simulink model "scalar_processor"  (Simulink 7.4)
settings: Solver=ode45  StartTime=0.0  StopTime=10.0  RelTol=1e-3
undefined symbols (not defined in the file): AS_ABS, CT_NONE, CT_S32, CT_U32
libraries: xbsIndex_r4 x517
(part 1 of 3)
settings Model: Creator=andryc  LastModifiedBy=andryc

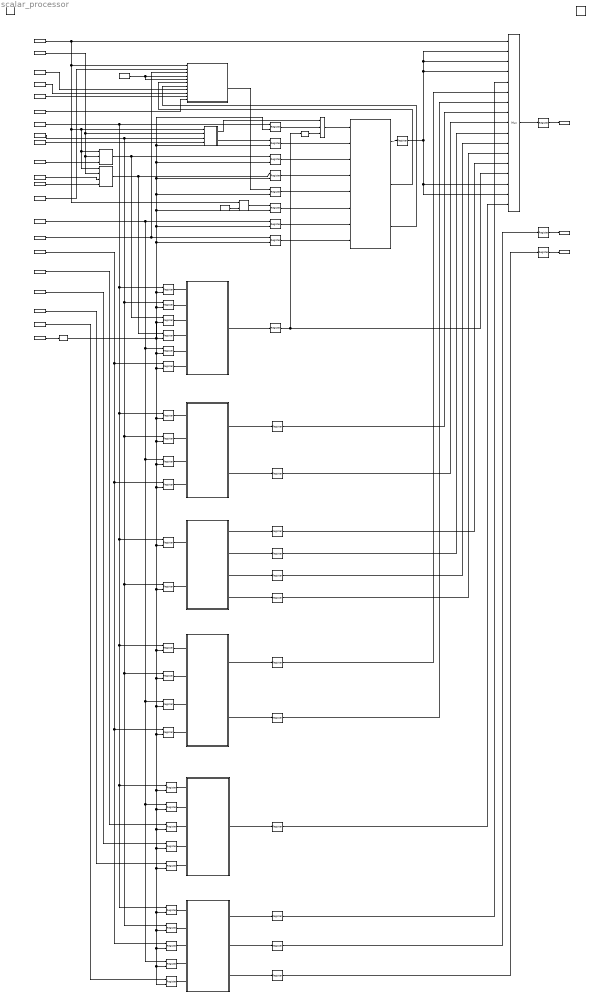
== system scalar_processor ==
  " System Generator" : xbsIndex_r4/ System Generator  Tag=genX  SystemSampleTime=-1  xilinxfamily=virtex5  part=xc5vlx50t  speed=-1  package=ff1136  synthesis_tool=XST  clock_wrapper=Clock Enables  directory=./ngc_netlist  testbench=off  simulink_period=1  sysclk_period=3.333333333  dcm_input_clock_period=10  incr_netlist=off  trim_vbits=Everywhere in SubSystem  dbl_ovrd=According to Block Masks  core_generation=According to Block Masks  run_coregen=off  deprecated_control=off  eval_field=0  block_type=sysgen
  Adder src_b select : Subsystem
  Boolean : Subsystem
  Constant : xbsIndex_r4/Constant  arith_type=Unsigned  const=3  n_bits=5  bin_pt=0  explicit_period=off  period=1  equ=P=C  opselect=C  inp2=PCIN>>17  opr=+  inp1=P  carry=CIN  dbl_ovrd=off  block_type=constant
  Constant1 : xbsIndex_r4/Constant  arith_type=Unsigned  const=0  n_bits=1  bin_pt=0  explicit_period=on  period=1  equ=P=C  opselect=C  inp2=PCIN>>17  opr=+  inp1=P  carry=CIN  dbl_ovrd=off  block_type=constant
  Convert : xbsIndex_r4/Convert  arith_type=Boolean  n_bits=16  bin_pt=14  quantization=Truncate  overflow=Wrap  en=off  latency=0  dbl_ovrd=off  pipeline=off  block_type=convert
  Convert Int to Int : Subsystem
  Convert1 : xbsIndex_r4/Convert  arith_type=Unsigned  n_bits=32  bin_pt=0  quantization=Truncate  overflow=Saturate  en=off  latency=0  dbl_ovrd=off  pipeline=off  block_type=convert
  Flag Registers : Subsystem
  Integer Add Subtract : Subsystem
  Integer Multiply 24-bit : Subsystem
  Min Max : Subsystem
  Mux : xbsIndex_r4/Mux  inputs=16  en=off  latency=0  precision=Full  arith_type=Unsigned  n_bits=16  bin_pt=14  quantization=Truncate  overflow=Wrap  dbl_ovrd=off  block_type=mux
  Mux1 : xbsIndex_r4/Mux  inputs=2  en=off  latency=0  precision=Full  arith_type=Unsigned  n_bits=16  bin_pt=14  quantization=Truncate  overflow=Wrap  dbl_ovrd=off  block_type=mux
  Register{,1..13,15..18,21..22,27..30,33..37,46..50} (34 alike) : xbsIndex_r4/Register  init=0  rst=off  en=on  dbl_ovrd=off  block_type=register
  Register{14,19..20,23..26,31..32,38..45} (17 alike) : xbsIndex_r4/Register  init=0  rst=off  en=off  dbl_ovrd=off  block_type=register
  Relational : xbsIndex_r4/Relational  mode=a=b  en=off  latency=0  dbl_ovrd=off  block_type=relational
  Resource Estimator : xbsIndex_r4/Resource Estimator  Tag=resEstTag  Slices=0  FFs=0  BRAMs=0  LUTs=0  IOBs=0  EBMs=0  TBUFs=0  xl_use_estimator_area=off  est_options=Estimate  block_type=resource_estimator
      settings: AttributesFormatString=Resource\nEstimator
  Shift Logical : Subsystem
  Subsystem : Subsystem
  Subsystem1 : Subsystem
  abs_saturate_in : xbsIndex_r4/Gateway In  arith_type=Unsigned  n_bits=2  bin_pt=0  quantization=Truncate  overflow=Saturate  period=1  dbl_ovrd=off  timing_constraint=None  locs_specified=off  LOCs={}  hdl_port=on  block_type=gatewayin
      settings: infoedit="Gateway in block.  Converts inputs of type Simulink integer, double and fixed point to  Xilinx fixed point type.<br><br>Hardware notes:  In hardware these blocks become top level input ports."
  alu_opcode_type_in : xbsIndex_r4/Gateway In  arith_type=Unsigned  n_bits=4  bin_pt=0  quantization=Truncate  overflow=Saturate  period=1  dbl_ovrd=off  timing_constraint=None  locs_specified=off  LOCs={}  hdl_port=on  block_type=gatewayin
      settings: infoedit="Gateway in block.  Converts inputs of type Simulink integer, double and fixed point to  Xilinx fixed point type.<br><br>Hardware notes:  In hardware these blocks become top level input ports."
  cvt_neg_in : xbsIndex_r4/Gateway In  arith_type=Unsigned  n_bits=1  bin_pt=0  quantization=Truncate  overflow=Saturate  period=1  dbl_ovrd=off  timing_constraint=None  locs_specified=off  LOCs={}  hdl_port=on  block_type=gatewayin
      settings: infoedit="Gateway in block.  Converts inputs of type Simulink integer, double and fixed point to  Xilinx fixed point type.<br><br>Hardware notes:  In hardware these blocks become top level input ports."
  cvt_type_in : xbsIndex_r4/Gateway In  arith_type=Unsigned  n_bits=3  bin_pt=0  quantization=Truncate  overflow=Saturate  period=1  dbl_ovrd=off  timing_constraint=None  locs_specified=off  LOCs={}  hdl_port=on  block_type=gatewayin
      settings: infoedit="Gateway in block.  Converts inputs of type Simulink integer, double and fixed point to  Xilinx fixed point type.<br><br>Hardware notes:  In hardware these blocks become top level input ports."
  en : xbsIndex_r4/Gateway In  arith_type=Unsigned  n_bits=1  bin_pt=0  quantization="Round  (unbiased: +/- Inf)"  overflow=Saturate  period=1  dbl_ovrd=off  timing_constraint=None  locs_specified=off  LOCs={}  hdl_port=on  block_type=gatewayin
      settings: infoedit="Gateway in block.  Converts inputs of type Simulink integer, double and fixed point to  Xilinx fixed point type.<br><br>Hardware notes:  In hardware these blocks become top level input ports."
  instr_marker_type_in : xbsIndex_r4/Gateway In  arith_type=Unsigned  n_bits=4  bin_pt=0  quantization=Truncate  overflow=Saturate  period=1  dbl_ovrd=off  timing_constraint=None  locs_specified=off  LOCs={}  hdl_port=on  block_type=gatewayin
      settings: infoedit="Gateway in block.  Converts inputs of type Simulink integer, double and fixed point to  Xilinx fixed point type.<br><br>Hardware notes:  In hardware these blocks become top level input ports."
  is_signed_in : xbsIndex_r4/Gateway In  arith_type=Unsigned  n_bits=1  bin_pt=0  quantization=Truncate  overflow=Saturate  period=1  dbl_ovrd=off  timing_constraint=None  locs_specified=off  LOCs={}  hdl_port=on  block_type=gatewayin
      settings: infoedit="Gateway in block.  Converts inputs of type Simulink integer, double and fixed point to  Xilinx fixed point type.<br><br>Hardware notes:  In hardware these blocks become top level input ports."
  pred_flag_carry_in : xbsIndex_r4/Gateway In  arith_type=Unsigned  n_bits=1  bin_pt=0  quantization=Truncate  overflow=Saturate  period=1  dbl_ovrd=off  timing_constraint=None  locs_specified=off  LOCs={}  hdl_port=on  block_type=gatewayin
      settings: infoedit="Gateway in block.  Converts inputs of type Simulink integer, double and fixed point to  Xilinx fixed point type.<br><br>Hardware notes:  In hardware these blocks become top level input ports."
  pred_flag_overflow_in : xbsIndex_r4/Gateway In  arith_type=Unsigned  n_bits=1  bin_pt=0  quantization=Truncate  overflow=Saturate  period=1  dbl_ovrd=off  timing_constraint=None  locs_specified=off  LOCs={}  hdl_port=on  block_type=gatewayin
      settings: infoedit="Gateway in block.  Converts inputs of type Simulink integer, double and fixed point to  Xilinx fixed point type.<br><br>Hardware notes:  In hardware these blocks become top level input ports."
  pred_flag_sign_in : xbsIndex_r4/Gateway In  arith_type=Unsigned  n_bits=1  bin_pt=0  quantization=Truncate  overflow=Saturate  period=1  dbl_ovrd=off  timing_constraint=None  locs_specified=off  LOCs={}  hdl_port=on  block_type=gatewayin
      settings: infoedit="Gateway in block.  Converts inputs of type Simulink integer, double and fixed point to  Xilinx fixed point type.<br><br>Hardware notes:  In hardware these blocks become top level input ports."
  pred_flag_sign_out : xbsIndex_r4/Gateway Out  hdl_port=on  timing_constraint=None  locs_specified=off  LOCs={}  block_type=gatewayout
      settings: infoedit="Gateway out block.  Converts Xilinx fixed point inputs into ouputs of type Simulink integer, double, or fixed point.<br><br>Hardware notes:  In hardware these blocks become top level output ports or are discarded, depending on how they are configured."
  pred_flag_zero_in : xbsIndex_r4/Gateway In  arith_type=Unsigned  n_bits=1  bin_pt=0  quantization=Truncate  overflow=Saturate  period=1  dbl_ovrd=off  timing_constraint=None  locs_specified=off  LOCs={}  hdl_port=on  block_type=gatewayin
      settings: infoedit="Gateway in block.  Converts inputs of type Simulink integer, double and fixed point to  Xilinx fixed point type.<br><br>Hardware notes:  In hardware these blocks become top level input ports."
  pred_flag_zero_out : xbsIndex_r4/Gateway Out  hdl_port=on  timing_constraint=None  locs_specified=off  LOCs={}  block_type=gatewayout
      settings: infoedit="Gateway out block.  Converts Xilinx fixed point inputs into ouputs of type Simulink integer, double, or fixed point.<br><br>Hardware notes:  In hardware these blocks become top level output ports or are discarded, depending on how they are configured."
  result_out : xbsIndex_r4/Gateway Out  hdl_port=on  timing_constraint=None  locs_specified=off  LOCs={}  block_type=gatewayout
      settings: infoedit="Gateway out block.  Converts Xilinx fixed point inputs into ouputs of type Simulink integer, double, or fixed point.<br><br>Hardware notes:  In hardware these blocks become top level output ports or are discarded, depending on how they are configured."
  saturate_in : xbsIndex_r4/Gateway In  arith_type=Unsigned  n_bits=1  bin_pt=0  quantization=Truncate  overflow=Saturate  period=1  dbl_ovrd=off  timing_constraint=None  locs_specified=off  LOCs={}  hdl_port=on  block_type=gatewayin
      settings: infoedit="Gateway in block.  Converts inputs of type Simulink integer, double and fixed point to  Xilinx fixed point type.<br><br>Hardware notes:  In hardware these blocks become top level input ports."
  set_cond_in : xbsIndex_r4/Gateway In  arith_type=Unsigned  n_bits=3  bin_pt=0  quantization=Truncate  overflow=Saturate  period=1  dbl_ovrd=off  timing_constraint=None  locs_specified=off  LOCs={}  hdl_port=on  block_type=gatewayin
      settings: infoedit="Gateway in block.  Converts inputs of type Simulink integer, double and fixed point to  Xilinx fixed point type.<br><br>Hardware notes:  In hardware these blocks become top level input ports."
  src_1_in : xbsIndex_r4/Gateway In  arith_type=Unsigned  n_bits=32  bin_pt=0  quantization=Truncate  overflow=Saturate  period=1  dbl_ovrd=off  timing_constraint=None  locs_specified=off  LOCs={}  hdl_port=on  block_type=gatewayin
      settings: infoedit="Gateway in block.  Converts inputs of type Simulink integer, double and fixed point to  Xilinx fixed point type.<br><br>Hardware notes:  In hardware these blocks become top level input ports."
  src_1_neg_in : xbsIndex_r4/Gateway In  arith_type=Unsigned  n_bits=1  bin_pt=0  quantization=Truncate  overflow=Saturate  period=1  dbl_ovrd=off  timing_constraint=None  locs_specified=off  LOCs={}  hdl_port=on  block_type=gatewayin
      settings: infoedit="Gateway in block.  Converts inputs of type Simulink integer, double and fixed point to  Xilinx fixed point type.<br><br>Hardware notes:  In hardware these blocks become top level input ports."
  src_2_in : xbsIndex_r4/Gateway In  arith_type=Unsigned  n_bits=32  bin_pt=0  quantization=Truncate  overflow=Saturate  period=1  dbl_ovrd=off  timing_constraint=None  locs_specified=off  LOCs={}  hdl_port=on  block_type=gatewayin
      settings: infoedit="Gateway in block.  Converts inputs of type Simulink integer, double and fixed point to  Xilinx fixed point type.<br><br>Hardware notes:  In hardware these blocks become top level input ports."
  src_2_neg_in : xbsIndex_r4/Gateway In  arith_type=Unsigned  n_bits=1  bin_pt=0  quantization=Truncate  overflow=Saturate  period=1  dbl_ovrd=off  timing_constraint=None  locs_specified=off  LOCs={}  hdl_port=on  block_type=gatewayin
      settings: infoedit="Gateway in block.  Converts inputs of type Simulink integer, double and fixed point to  Xilinx fixed point type.<br><br>Hardware notes:  In hardware these blocks become top level input ports."
  src_3_in : xbsIndex_r4/Gateway In  arith_type=Unsigned  n_bits=32  bin_pt=0  quantization=Truncate  overflow=Saturate  period=1  dbl_ovrd=off  timing_constraint=None  locs_specified=off  LOCs={}  hdl_port=on  block_type=gatewayin
      settings: infoedit="Gateway in block.  Converts inputs of type Simulink integer, double and fixed point to  Xilinx fixed point type.<br><br>Hardware notes:  In hardware these blocks become top level input ports."
  src_3_neg_in : xbsIndex_r4/Gateway In  arith_type=Unsigned  n_bits=1  bin_pt=0  quantization=Truncate  overflow=Saturate  period=1  dbl_ovrd=off  timing_constraint=None  locs_specified=off  LOCs={}  hdl_port=on  block_type=gatewayin
      settings: infoedit="Gateway in block.  Converts inputs of type Simulink integer, double and fixed point to  Xilinx fixed point type.<br><br>Hardware notes:  In hardware these blocks become top level input ports."
  src_a_neg select : Subsystem
  use_carry_in : xbsIndex_r4/Gateway In  arith_type=Unsigned  n_bits=1  bin_pt=0  quantization=Truncate  overflow=Saturate  period=1  dbl_ovrd=off  timing_constraint=None  locs_specified=off  LOCs={}  hdl_port=on  block_type=gatewayin
      settings: infoedit="Gateway in block.  Converts inputs of type Simulink integer, double and fixed point to  Xilinx fixed point type.<br><br>Hardware notes:  In hardware these blocks become top level input ports."
  w32_in : xbsIndex_r4/Gateway In  arith_type=Unsigned  n_bits=1  bin_pt=0  quantization=Truncate  overflow=Saturate  period=1  dbl_ovrd=off  timing_constraint=None  locs_specified=off  LOCs={}  hdl_port=on  block_type=gatewayin
      settings: infoedit="Gateway in block.  Converts inputs of type Simulink integer, double and fixed point to  Xilinx fixed point type.<br><br>Hardware notes:  In hardware these blocks become top level input ports."
  wires:
  Register1/1 -> Integer Add Subtract/2(b)
  Register2/1 -> Integer Add Subtract/3(a_neg)
  Register3/1 -> Integer Add Subtract/4(b_neg)
  Register4/1 -> Integer Add Subtract/5(cin)
  Register5/1 -> Integer Add Subtract/6(sub_en)
  Register6/1 -> Integer Add Subtract/7(w32)
  Register7/1 -> Integer Add Subtract/8(saturate)
  src_1_in/1 -> Register/1, Register8/1, Register15/1, Register21/1, Register27/1, Register33/1, Register46/1
  Flag Registers/3(carry_out) -> Register4/1
  use_carry_in/1 -> Flag Registers/2(use_cin)
  w32_in/1 -> Register6/1, Register12/1, Register17/1, Register29/1, Register34/1, Register49/1
  saturate_in/1 -> Register7/1, Flag Registers/3(sat)
  Constant/1 -> Relational/2
  alu_opcode_type_in/1 -> Relational/1, Adder src_b select/1(opcode), src_a_neg select/1(opcode), Subsystem1/1(opcode), Flag Registers/1(opcode), Mux/1
  Relational/1 -> Register5/1
  Integer Add Subtract/2(cout) -> Flag Registers/6(carry_in)
  Integer Add Subtract/3(overflow) -> Flag Registers/7(overflow_in)
  Adder src_b select/2(b) -> Register1/1
  Adder src_b select/1(is_mad) -> Mux1/1
  Mux1/1 -> Integer Add Subtract/1(a)
  instr_marker_type_in/1 -> Adder src_b select/2(marker), src_a_neg select/2(marker), Subsystem1/2(marker)
  src_2_in/1 -> Adder src_b select/3(src2), Register9/1, Register16/1, Register22/1, Register28/1, Register47/1
  src_3_in/1 -> Adder src_b select/4(src3)
  src_a_neg select/1(a_neg) -> Register2/1, Register10/1
  src_1_neg_in/1 -> src_a_neg select/3(src1_neg)
  Subsystem1/1(b_neg) -> Register3/1, Register11/1
  src_2_neg_in/1 -> Subsystem1/3(src2_neg)
  src_3_neg_in/1 -> Subsystem1/4(src3_neg)
  Register8/1 -> Integer Multiply 24-bit/1(a)
  Register9/1 -> Integer Multiply 24-bit/2(b)
  is_signed_in/1 -> Register13/1, Register18/1, Register30/1, Register48/1
  Register10/1 -> Integer Multiply 24-bit/3(a_neg)
  Register11/1 -> Integer Multiply 24-bit/4(b_neg)
  Register12/1 -> Integer Multiply 24-bit/5(w32)
  Register13/1 -> Integer Multiply 24-bit/6(is_signed)
  pred_flag_overflow_in/1 -> Flag Registers/11(pred_overflow_in)
  pred_flag_carry_in/1 -> Flag Registers/10(pred_carry_in)
  pred_flag_sign_in/1 -> Flag Registers/9(pred_sign_in)
  Register/1 -> Mux1/2
  Integer Multiply 24-bit/1(result) -> Register14/1
  Register14/1 -> Mux/14, Convert1/1
  pred_flag_zero_in/1 -> Flag Registers/8(pred_zero_in)
  Register15/1 -> Shift Logical/1(a)
  Register16/1 -> Shift Logical/2(b)
  Register17/1 -> Shift Logical/3(w32)
  Register18/1 -> Shift Logical/4(is_signed)
  Shift Logical/1(shift_left) -> Register19/1
  Shift Logical/2(shift_right) -> Register20/1
  Register21/1 -> Boolean/1(a)
  Register22/1 -> Boolean/2(b)
  Boolean/1(neg) -> Register23/1
  Boolean/2(and) -> Register24/1
  Boolean/3(or) -> Register25/1
  Boolean/4(xor) -> Register26/1
  Register27/1 -> Min Max/1(a)
  Register28/1 -> Min Max/2(b)
  Register29/1 -> Min Max/3(w32)
  Register30/1 -> Min Max/4(is_signed)
  Min Max/1(min) -> Register31/1
  Min Max/2(max) -> Register32/1
  Register33/1 -> Convert Int to Int/1(a)
  Register34/1 -> Convert Int to Int/2(w32)
  Register35/1 -> Convert Int to Int/3(cvt_type)
  Register36/1 -> Convert Int to Int/4(abs_sat)
  Register37/1 -> Convert Int to Int/5(neg)
  Convert Int to Int/1(result) -> Register38/1
  cvt_type_in/1 -> Register35/1
  abs_saturate_in/1 -> Register36/1
  cvt_neg_in/1 -> Register37/1
  en/1 -> Convert/1
  Mux/1 -> Register40/1
  Integer Add Subtract/1(result) -> Register39/1
  Register39/1 -> Mux/2, Mux/3, Mux/4, Mux/15, Mux/16
  Register31/1 -> Mux/6
  Register32/1 -> Mux/7
  Register19/1 -> Mux/8
  Register20/1 -> Mux/9
  Register24/1 -> Mux/10
  Register25/1 -> Mux/11
  Register26/1 -> Mux/12
  Register23/1 -> Mux/13
  Register38/1 -> Mux/17
  Register40/1 -> result_out/1
  Register41/1 -> pred_flag_zero_out/1
  Register42/1 -> pred_flag_sign_out/1
  Subsystem/1(result) -> Register43/1
  Subsystem/2(sign) -> Register44/1
  Subsystem/3(zero) -> Register45/1
  Register46/1 -> Subsystem/1(a)
  Register47/1 -> Subsystem/2(b)
  Register48/1 -> Subsystem/3(is_signed)
  Register49/1 -> Subsystem/4(w32)
  Register50/1 -> Subsystem/5(set_cond)
  set_cond_in/1 -> Register50/1
  Register43/1 -> Mux/5
  Register44/1 -> Register42/1
  Register45/1 -> Register41/1
  Constant1/1 -> Flag Registers/4(zero_in), Flag Registers/5(sign_in)
  Convert/1 -> Register10/2, Register9/2, Register8/2, Register7/2, Register6/2, Register5/2, Register4/2, Register3/2, Register2/2, Register1/2, Register/2, Register11/2, Register12/2, Register13/2, Register15/2, Register16/2, Register17/2, Register18/2, Register21/2, Register22/2, Register27/2, Register28/2, Register29/2, Register30/2, Register33/2, Register34/2, Register35/2, Register36/2, Register37/2, Register46/2, Register47/2, Register48/2, Register49/2, Register50/2
  Convert1/1 -> Mux1/3

== system scalar_processor/Adder src_b select ==
  opcode : Inport
  marker : Inport  Port=2
  src2 : Inport  Port=3
  src3 : Inport  Port=4
  Constant1 : xbsIndex_r4/Constant  arith_type=Unsigned  const=0  n_bits=4  bin_pt=0  explicit_period=off  period=1  equ=P=C  opselect=C  inp2=PCIN>>17  opr=+  inp1=P  carry=CIN  dbl_ovrd=off  block_type=constant
  Constant2 : xbsIndex_r4/Constant  arith_type=Unsigned  const=1  n_bits=4  bin_pt=0  explicit_period=off  period=1  equ=P=C  opselect=C  inp2=PCIN>>17  opr=+  inp1=P  carry=CIN  dbl_ovrd=off  block_type=constant
  Constant3 : xbsIndex_r4/Constant  arith_type=Unsigned  const=2  n_bits=4  bin_pt=0  explicit_period=off  period=1  equ=P=C  opselect=C  inp2=PCIN>>17  opr=+  inp1=P  carry=CIN  dbl_ovrd=off  block_type=constant
  Logical : xbsIndex_r4/Logical  logical_function=OR  inputs=4  en=off  latency=0  precision=Full  arith_type=Unsigned  n_bits=16  bin_pt=0  align_bp=on  dbl_ovrd=off  block_type=logical
  Mux2 : xbsIndex_r4/Mux  inputs=2  en=off  latency=0  precision=Full  arith_type=Unsigned  n_bits=16  bin_pt=14  quantization=Truncate  overflow=Wrap  dbl_ovrd=off  block_type=mux
  Relational1 : xbsIndex_r4/Relational  mode=a=b  en=off  latency=0  dbl_ovrd=off  block_type=relational
  Relational2 : xbsIndex_r4/Relational  mode=a=b  en=off  latency=0  dbl_ovrd=off  block_type=relational
  Relational3 : xbsIndex_r4/Relational  mode=a=b  en=off  latency=0  dbl_ovrd=off  block_type=relational
  Subsystem2 : Subsystem
  is_mad : Outport
  b : Outport  Port=2
  wires:
  Constant1/1 -> Relational1/2
  Constant2/1 -> Relational2/2
  Subsystem2/1(is_imad) -> Logical/1, is_mad/1
  Relational1/1 -> Logical/2
  Relational2/1 -> Logical/3
  Logical/1 -> Mux2/1
  opcode/1 -> Subsystem2/1(opcode)
  marker/1 -> Relational1/1, Relational2/1, Relational3/1
  src2/1 -> Mux2/2
  Mux2/1 -> b/1
  src3/1 -> Mux2/3
  Constant3/1 -> Relational3/2
  Relational3/1 -> Logical/4

== system scalar_processor/Boolean ==
  a : Inport
  b : Inport  Port=2
  Logical : xbsIndex_r4/Logical  logical_function=AND  inputs=2  en=off  latency=0  precision=Full  arith_type=Unsigned  n_bits=16  bin_pt=0  align_bp=on  dbl_ovrd=off  block_type=logical
  Logical1 : xbsIndex_r4/Logical  logical_function=OR  inputs=2  en=off  latency=0  precision=Full  arith_type=Unsigned  n_bits=16  bin_pt=0  align_bp=on  dbl_ovrd=off  block_type=logical
  Logical2 : xbsIndex_r4/Logical  logical_function=XOR  inputs=2  en=off  latency=0  precision=Full  arith_type=Unsigned  n_bits=16  bin_pt=0  align_bp=on  dbl_ovrd=off  block_type=logical
  Negate : xbsIndex_r4/Negate  precision=Full  arith_type="Signed  (2's comp)"  n_bits=16  bin_pt=14  quantization=Truncate  overflow=Wrap  en=off  latency=0  dbl_ovrd=off  block_type=negate
  neg : Outport
  and : Outport  Port=2
  or : Outport  Port=3
  xor : Outport  Port=4
  wires:
  a/1 -> Negate/1, Logical/1, Logical1/1, Logical2/1
  Negate/1 -> neg/1
  Logical/1 -> and/1
  b/1 -> Logical/2, Logical1/2, Logical2/2
  Logical1/1 -> or/1
  Logical2/1 -> xor/1

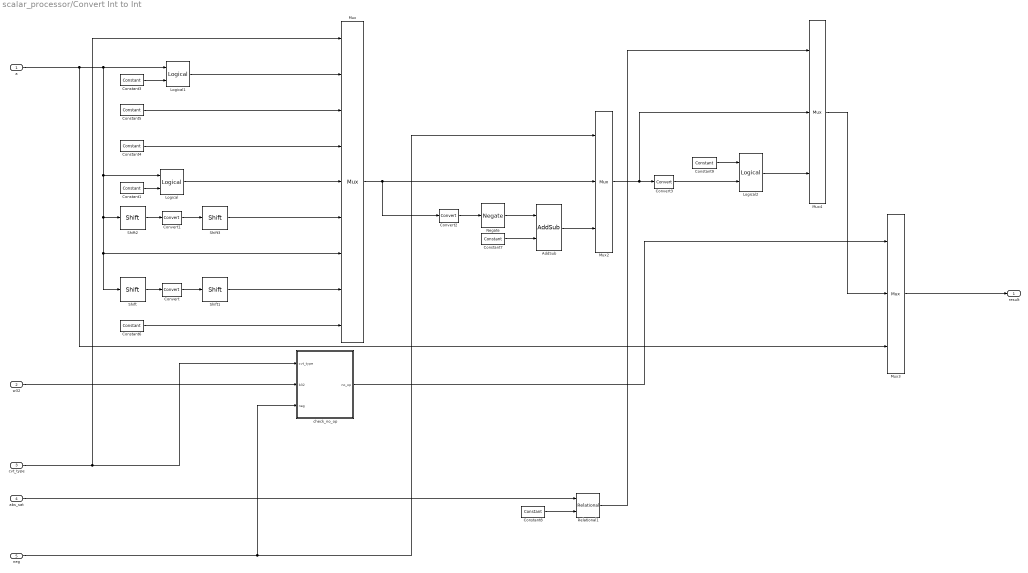
== system scalar_processor/Convert Int to Int ==
  a : Inport
  w32 : Inport  Port=2
  cvt_type : Inport  Port=3
  abs_sat : Inport  Port=4
  neg : Inport  Port=5
  AddSub : xbsIndex_r4/AddSub  mode=Addition  use_carryin=off  use_carryout=off  en=off  latency=0  precision=User Defined  arith_type=Unsigned  n_bits=32  bin_pt=0  quantization=Truncate  overflow=Saturate  dbl_ovrd=off  use_behavioral_HDL=off  hw_selection=Fabric  pipelined=off  block_type=addsub
      settings: block_version=12.2
  Constant1 : xbsIndex_r4/Constant  arith_type=Unsigned  const=255  n_bits=32  bin_pt=0  explicit_period=off  period=1  equ=P=C  opselect=C  inp2=PCIN>>17  opr=+  inp1=P  carry=CIN  dbl_ovrd=off  block_type=constant
      settings: block_version=12.2
  Constant3 : xbsIndex_r4/Constant  arith_type=Unsigned  const=65535  n_bits=32  bin_pt=0  explicit_period=off  period=1  equ=P=C  opselect=C  inp2=PCIN>>17  opr=+  inp1=P  carry=CIN  dbl_ovrd=off  block_type=constant
      settings: block_version=12.2
  Constant4 : xbsIndex_r4/Constant  arith_type=Unsigned  const=0  n_bits=32  bin_pt=0  explicit_period=off  period=1  equ=P=C  opselect=C  inp2=PCIN>>17  opr=+  inp1=P  carry=CIN  dbl_ovrd=off  block_type=constant
      settings: block_version=12.2
  Constant5 : xbsIndex_r4/Constant  arith_type=Unsigned  const=0  n_bits=32  bin_pt=0  explicit_period=off  period=1  equ=P=C  opselect=C  inp2=PCIN>>17  opr=+  inp1=P  carry=CIN  dbl_ovrd=off  block_type=constant
      settings: block_version=12.2
  Constant6 : xbsIndex_r4/Constant  arith_type=Unsigned  const=0  n_bits=32  bin_pt=0  explicit_period=off  period=1  equ=P=C  opselect=C  inp2=PCIN>>17  opr=+  inp1=P  carry=CIN  dbl_ovrd=off  block_type=constant
      settings: block_version=12.2
  Constant7 : xbsIndex_r4/Constant  arith_type=Unsigned  const=1  n_bits=32  bin_pt=0  explicit_period=off  period=1  equ=P=C  opselect=C  inp2=PCIN>>17  opr=+  inp1=P  carry=CIN  dbl_ovrd=off  block_type=constant
      settings: block_version=12.2
  Constant8 : xbsIndex_r4/Constant  arith_type=Unsigned  const=AS_ABS  n_bits=2  bin_pt=0  explicit_period=off  period=1  equ=P=C  opselect=C  inp2=PCIN>>17  opr=+  inp1=P  carry=CIN  dbl_ovrd=off  block_type=constant
      settings: block_version=12.2
  Constant9 : xbsIndex_r4/Constant  arith_type=Unsigned  const=2147483647  n_bits=32  bin_pt=0  explicit_period=off  period=1  equ=P=C  opselect=C  inp2=PCIN>>17  opr=+  inp1=P  carry=CIN  dbl_ovrd=off  block_type=constant
      settings: block_version=12.2
  Convert : xbsIndex_r4/Convert  arith_type="Signed  (2's comp)"  n_bits=32  bin_pt=0  quantization=Truncate  overflow=Saturate  en=off  latency=0  dbl_ovrd=off  pipeline=off  block_type=convert
      settings: block_version=12.2
  Convert1 : xbsIndex_r4/Convert  arith_type="Signed  (2's comp)"  n_bits=32  bin_pt=0  quantization=Truncate  overflow=Saturate  en=off  latency=0  dbl_ovrd=off  pipeline=off  block_type=convert
      settings: block_version=12.2
  Convert2 : xbsIndex_r4/Convert  arith_type=Unsigned  n_bits=32  bin_pt=0  quantization=Truncate  overflow=Saturate  en=off  latency=0  dbl_ovrd=off  pipeline=off  block_type=convert
      settings: block_version=12.2
  Convert3 : xbsIndex_r4/Convert  arith_type="Signed  (2's comp)"  n_bits=32  bin_pt=0  quantization=Truncate  overflow=Saturate  en=off  latency=0  dbl_ovrd=off  pipeline=off  block_type=convert
      settings: block_version=12.2
  Logical : xbsIndex_r4/Logical  logical_function=AND  inputs=2  en=off  latency=0  precision=User Defined  arith_type=Unsigned  n_bits=32  bin_pt=0  align_bp=on  dbl_ovrd=off  block_type=logical
      settings: block_version=12.2
  Logical1 : xbsIndex_r4/Logical  logical_function=AND  inputs=2  en=off  latency=0  precision=User Defined  arith_type=Unsigned  n_bits=32  bin_pt=0  align_bp=on  dbl_ovrd=off  block_type=logical
      settings: block_version=12.2
  Logical2 : xbsIndex_r4/Logical  logical_function=AND  inputs=2  en=off  latency=0  precision=User Defined  arith_type="Signed  (2's comp)"  n_bits=32  bin_pt=0  align_bp=on  dbl_ovrd=off  block_type=logical
      settings: block_version=12.2
  Mux : xbsIndex_r4/Mux  inputs=8  en=off  latency=0  precision=User Defined  arith_type=Unsigned  n_bits=32  bin_pt=0  quantization=Truncate  overflow=Saturate  dbl_ovrd=off  block_type=mux
      settings: block_version=12.2
  Mux2 : xbsIndex_r4/Mux  inputs=2  en=off  latency=0  precision=User Defined  arith_type=Unsigned  n_bits=32  bin_pt=0  quantization=Truncate  overflow=Saturate  dbl_ovrd=off  block_type=mux
      settings: block_version=12.2
  Mux3 : xbsIndex_r4/Mux  inputs=2  en=off  latency=0  precision=User Defined  arith_type=Unsigned  n_bits=32  bin_pt=0  quantization=Truncate  overflow=Saturate  dbl_ovrd=off  block_type=mux
      settings: block_version=12.2
  Mux4 : xbsIndex_r4/Mux  inputs=2  en=off  latency=0  precision=User Defined  arith_type=Unsigned  n_bits=32  bin_pt=0  quantization=Truncate  overflow=Saturate  dbl_ovrd=off  block_type=mux
      settings: block_version=12.2
  Negate : xbsIndex_r4/Negate  precision=Full  arith_type="Signed  (2's comp)"  n_bits=16  bin_pt=14  quantization=Truncate  overflow=Wrap  en=off  latency=0  dbl_ovrd=off  block_type=negate
      settings: block_version=12.2
  Relational1 : xbsIndex_r4/Relational  mode=a=b  en=off  latency=0  dbl_ovrd=off  block_type=relational
      settings: block_version=12.2
  Shift : xbsIndex_r4/Shift  shift_dir=Left  shift_bits=24  en=off  latency=0  precision=User Defined  arith_type=Unsigned  n_bits=32  bin_pt=14  quantization=Truncate  overflow=Saturate  dbl_ovrd=off  block_type=shift
      settings: block_version=12.2
  Shift1 : xbsIndex_r4/Shift  shift_dir=Right  shift_bits=24  en=off  latency=0  precision=User Defined  arith_type="Signed  (2's comp)"  n_bits=32  bin_pt=0  quantization=Truncate  overflow=Saturate  dbl_ovrd=off  block_type=shift
      settings: block_version=12.2
  Shift2 : xbsIndex_r4/Shift  shift_dir=Left  shift_bits=16  en=off  latency=0  precision=User Defined  arith_type=Unsigned  n_bits=32  bin_pt=14  quantization=Truncate  overflow=Saturate  dbl_ovrd=off  block_type=shift
      settings: block_version=12.2
  Shift3 : xbsIndex_r4/Shift  shift_dir=Right  shift_bits=16  en=off  latency=0  precision=User Defined  arith_type="Signed  (2's comp)"  n_bits=32  bin_pt=0  quantization=Truncate  overflow=Saturate  dbl_ovrd=off  block_type=shift
      settings: block_version=12.2
  check_no_op : Subsystem
  result : Outport
  wires:
  neg/1 -> check_no_op/3(neg), Mux2/1
  cvt_type/1 -> Mux/1, check_no_op/1(cvt_type)
  Constant1/1 -> Logical/2
  Shift/1 -> Convert/1
  Convert/1 -> Shift1/1
  Constant3/1 -> Logical1/2
  Shift2/1 -> Convert1/1
  Convert1/1 -> Shift3/1
  Constant4/1 -> Mux/4
  Logical/1 -> Mux/5
  Shift1/1 -> Mux/8
  Logical1/1 -> Mux/2
  Shift3/1 -> Mux/6
  Constant5/1 -> Mux/3
  Constant6/1 -> Mux/9
  a/1 -> Logical1/1, Logical/1, Shift2/1, Mux/7, Shift/1, Mux3/3
  Convert2/1 -> Negate/1
  Negate/1 -> AddSub/1
  Constant7/1 -> AddSub/2
  AddSub/1 -> Mux2/3
  Mux/1 -> Mux2/2, Convert2/1
  Constant8/1 -> Relational1/2
  Relational1/1 -> Mux4/1
  Mux2/1 -> Convert3/1, Mux4/2
  Constant9/1 -> Logical2/1
  check_no_op/1(no_op) -> Mux3/1
  Mux4/1 -> Mux3/2
  Logical2/1 -> Mux4/3
  Convert3/1 -> Logical2/2
  Mux3/1 -> result/1
  w32/1 -> check_no_op/2(b32)
  abs_sat/1 -> Relational1/1

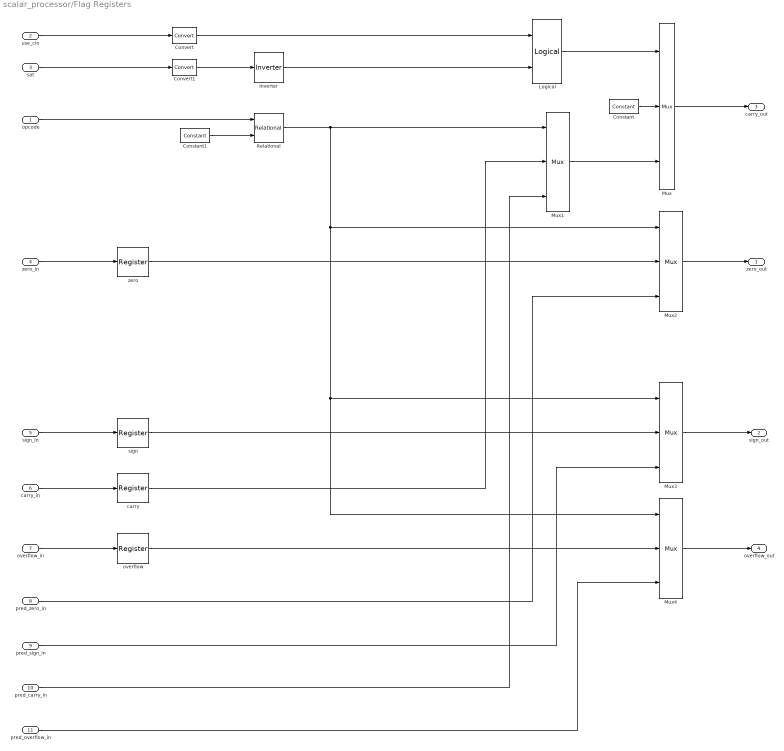
== system scalar_processor/Flag Registers ==
  opcode : Inport
  use_cin : Inport  Port=2
  sat : Inport  Port=3
  zero_in : Inport  Port=4
  sign_in : Inport  Port=5
  carry_in : Inport  Port=6
  overflow_in : Inport  Port=7
  pred_zero_in : Inport  Port=8
  pred_sign_in : Inport  Port=9
  pred_carry_in : Inport  Port=10
  pred_overflow_in : Inport  Port=11
  Constant : xbsIndex_r4/Constant  arith_type=Unsigned  const=0  n_bits=1  bin_pt=0  explicit_period=off  period=1  equ=P=C  opselect=C  inp2=PCIN>>17  opr=+  inp1=P  carry=CIN  dbl_ovrd=off  block_type=constant
  Constant1 : xbsIndex_r4/Constant  arith_type=Unsigned  const=1  n_bits=4  bin_pt=0  explicit_period=off  period=1  equ=P=C  opselect=C  inp2=PCIN>>17  opr=+  inp1=P  carry=CIN  dbl_ovrd=off  block_type=constant
  Convert : xbsIndex_r4/Convert  arith_type=Boolean  n_bits=16  bin_pt=14  quantization=Truncate  overflow=Wrap  en=off  latency=0  dbl_ovrd=off  pipeline=off  block_type=convert
  Convert1 : xbsIndex_r4/Convert  arith_type=Boolean  n_bits=16  bin_pt=14  quantization=Truncate  overflow=Wrap  en=off  latency=0  dbl_ovrd=off  pipeline=off  block_type=convert
  Inverter : xbsIndex_r4/Inverter  en=off  latency=0  dbl_ovrd=off  block_type=inv
  Logical : xbsIndex_r4/Logical  logical_function=AND  inputs=2  en=off  latency=0  precision=Full  arith_type=Unsigned  n_bits=16  bin_pt=0  align_bp=on  dbl_ovrd=off  block_type=logical
  Mux{,1..4} (5 alike) : xbsIndex_r4/Mux  inputs=2  en=off  latency=0  precision=Full  arith_type=Unsigned  n_bits=16  bin_pt=14  quantization=Truncate  overflow=Wrap  dbl_ovrd=off  block_type=mux
  Relational : xbsIndex_r4/Relational  mode=a=b  en=off  latency=0  dbl_ovrd=off  block_type=relational
  carry : xbsIndex_r4/Register  init=0  rst=off  en=off  dbl_ovrd=off  block_type=register
  overflow : xbsIndex_r4/Register  init=0  rst=off  en=off  dbl_ovrd=off  block_type=register
  sign : xbsIndex_r4/Register  init=0  rst=off  en=off  dbl_ovrd=off  block_type=register
  zero : xbsIndex_r4/Register  init=0  rst=off  en=off  dbl_ovrd=off  block_type=register
  zero_out : Outport
  sign_out : Outport  Port=2
  carry_out : Outport  Port=3
  overflow_out : Outport  Port=4
  wires:
  zero_in/1 -> zero/1
  sign_in/1 -> sign/1
  carry_in/1 -> carry/1
  overflow_in/1 -> overflow/1
  Constant1/1 -> Relational/2
  opcode/1 -> Relational/1
  Relational/1 -> Mux1/1, Mux2/1, Mux3/1, Mux4/1
  pred_carry_in/1 -> Mux1/3
  carry/1 -> Mux1/2
  Mux1/1 -> Mux/3
  Constant/1 -> Mux/2
  Logical/1 -> Mux/1
  use_cin/1 -> Convert/1
  Inverter/1 -> Logical/2
  Mux/1 -> carry_out/1
  zero/1 -> Mux2/2
  pred_zero_in/1 -> Mux2/3
  Mux2/1 -> zero_out/1
  Mux3/1 -> sign_out/1
  sign/1 -> Mux3/2
  pred_sign_in/1 -> Mux3/3
  overflow/1 -> Mux4/2
  Mux4/1 -> overflow_out/1
  pred_overflow_in/1 -> Mux4/3
  Convert/1 -> Logical/1
  sat/1 -> Convert1/1
  Convert1/1 -> Inverter/1

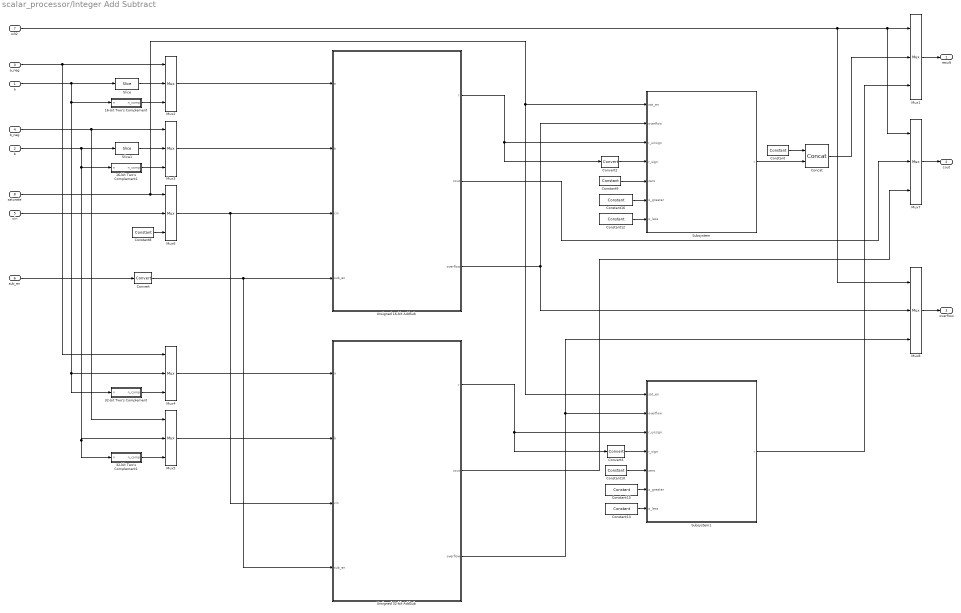
== system scalar_processor/Integer Add Subtract ==
  a : Inport
  b : Inport  Port=2
  a_neg : Inport  Port=3
  b_neg : Inport  Port=4
  cin : Inport  Port=5
  sub_en : Inport  Port=6
  w32 : Inport  Port=7
  saturate : Inport  Port=8
  16-bit Two's Complement : Subsystem
  16-bit Two's Complement1 : Subsystem
  32-bit Two's Complement : Subsystem
  32-bit Two's Complement1 : Subsystem
  Concat : xbsIndex_r4/Concat  num_inputs=2  dbl_ovrd=off  block_type=concat
  Constant : xbsIndex_r4/Constant  arith_type=Unsigned  const=0  n_bits=16  bin_pt=0  explicit_period=off  period=1  equ=P=C  opselect=C  inp2=PCIN>>17  opr=+  inp1=P  carry=CIN  dbl_ovrd=off  block_type=constant
  Constant10 : xbsIndex_r4/Constant  arith_type=Signed (2's comp)  const=0  n_bits=32  bin_pt=0  explicit_period=off  period=1  equ=P=C  opselect=C  inp2=PCIN>>17  opr=+  inp1=P  carry=CIN  dbl_ovrd=off  block_type=constant
  Constant12 : xbsIndex_r4/Constant  arith_type=Unsigned  const=32767  n_bits=16  bin_pt=0  explicit_period=off  period=1  equ=P=C  opselect=C  inp2=PCIN>>17  opr=+  inp1=P  carry=CIN  dbl_ovrd=off  block_type=constant
  Constant13 : xbsIndex_r4/Constant  arith_type=Unsigned  const=2147483647  n_bits=32  bin_pt=0  explicit_period=off  period=1  equ=P=C  opselect=C  inp2=PCIN>>17  opr=+  inp1=P  carry=CIN  dbl_ovrd=off  block_type=constant
  Constant15 : xbsIndex_r4/Constant  arith_type=Unsigned  const=2147483648  n_bits=32  bin_pt=0  explicit_period=off  period=1  equ=P=C  opselect=C  inp2=PCIN>>17  opr=+  inp1=P  carry=CIN  dbl_ovrd=off  block_type=constant
  Constant16 : xbsIndex_r4/Constant  arith_type=Unsigned  const=32768  n_bits=16  bin_pt=0  explicit_period=off  period=1  equ=P=C  opselect=C  inp2=PCIN>>17  opr=+  inp1=P  carry=CIN  dbl_ovrd=off  block_type=constant
  Constant8 : xbsIndex_r4/Constant  arith_type=Unsigned  const=0  n_bits=1  bin_pt=0  explicit_period=off  period=1  equ=P=C  opselect=C  inp2=PCIN>>17  opr=+  inp1=P  carry=CIN  dbl_ovrd=off  block_type=constant
  Constant9 : xbsIndex_r4/Constant  arith_type=Signed (2's comp)  const=0  n_bits=16  bin_pt=0  explicit_period=off  period=1  equ=P=C  opselect=C  inp2=PCIN>>17  opr=+  inp1=P  carry=CIN  dbl_ovrd=off  block_type=constant
  Convert : xbsIndex_r4/Convert  arith_type=Boolean  n_bits=16  bin_pt=14  quantization=Truncate  overflow=Wrap  en=off  latency=0  dbl_ovrd=off  pipeline=off  block_type=convert
  Convert2 : xbsIndex_r4/Convert  arith_type="Signed  (2's comp)"  n_bits=16  bin_pt=0  quantization=Truncate  overflow=Saturate  en=off  latency=0  dbl_ovrd=off  pipeline=off  block_type=convert
  Convert3 : xbsIndex_r4/Convert  arith_type="Signed  (2's comp)"  n_bits=32  bin_pt=0  quantization=Truncate  overflow=Saturate  en=off  latency=0  dbl_ovrd=off  pipeline=off  block_type=convert
  Mux{1..8} (8 alike) : xbsIndex_r4/Mux  inputs=2  en=off  latency=0  precision=Full  arith_type=Unsigned  n_bits=16  bin_pt=14  quantization=Truncate  overflow=Wrap  dbl_ovrd=off  block_type=mux
  Slice : xbsIndex_r4/Slice  nbits=16  boolean_output=off  mode=Lower Bit Location + Width  bit1=0  base1=MSB of Input  bit0=0  base0=LSB of Input  dbl_ovrd=off  block_type=slice
  Slice1 : xbsIndex_r4/Slice  nbits=16  boolean_output=off  mode=Lower Bit Location + Width  bit1=0  base1=MSB of Input  bit0=0  base0=LSB of Input  dbl_ovrd=off  block_type=slice
  Subsystem : Subsystem
  Subsystem1 : Subsystem
  Unsigned 16-bit AddSub : Subsystem
  Unsigned 32-bit AddSub : Subsystem
  result : Outport
  cout : Outport  Port=2
  overflow : Outport  Port=3
  wires:
  Convert/1 -> Unsigned 32-bit AddSub/4(sub_en), Unsigned 16-bit AddSub/4(sub_en)
  Mux2/1 -> Unsigned 16-bit AddSub/1(a)
  16-bit Two's Complement/1(n_comp) -> Mux2/3
  Slice/1 -> Mux2/2
  Mux3/1 -> Unsigned 16-bit AddSub/2(b)
  Slice1/1 -> Mux3/2
  16-bit Two's Complement1/1(n_comp) -> Mux3/3
  Mux4/1 -> Unsigned 32-bit AddSub/1(a)
  32-bit Two's Complement/1(n_comp) -> Mux4/3
  Mux5/1 -> Unsigned 32-bit AddSub/2(b)
  32-bit Two's Complement1/1(n_comp) -> Mux5/3
  Mux6/1 -> Unsigned 16-bit AddSub/3(cin), Unsigned 32-bit AddSub/3(cin)
  Constant8/1 -> Mux6/3
  Convert2/1 -> Subsystem/4(r_sign)
  Constant9/1 -> Subsystem/5(zero)
  Unsigned 16-bit AddSub/3(overflow) -> Subsystem/2(overflow), Mux8/2
  Constant12/1 -> Subsystem/7(o_less)
  Constant16/1 -> Subsystem/6(o_greater)
  Unsigned 16-bit AddSub/1(r) -> Convert2/1, Subsystem/3(r_unsign)
  Unsigned 32-bit AddSub/3(overflow) -> Subsystem1/2(overflow), Mux8/3
  Constant10/1 -> Subsystem1/5(zero)
  Convert3/1 -> Subsystem1/4(r_sign)
  Unsigned 32-bit AddSub/1(r) -> Convert3/1, Subsystem1/3(r_unsign)
  Constant15/1 -> Subsystem1/6(o_greater)
  Constant13/1 -> Subsystem1/7(o_less)
  Subsystem1/1(r) -> Mux1/3
  Mux1/1 -> result/1
  Mux7/1 -> cout/1
  Unsigned 16-bit AddSub/2(cout) -> Mux7/2
  Unsigned 32-bit AddSub/2(cout) -> Mux7/3
  Mux8/1 -> overflow/1
  w32/1 -> Mux1/1, Mux7/1, Mux8/1
  a_neg/1 -> Mux2/1, Mux4/1
  a/1 -> 16-bit Two's Complement/1(n), 32-bit Two's Complement/1(n), Mux4/2, Slice/1
  b_neg/1 -> Mux3/1, Mux5/1
  b/1 -> 32-bit Two's Complement1/1(n), Mux5/2, 16-bit Two's Complement1/1(n), Slice1/1
  saturate/1 -> Mux6/1, Subsystem/1(sat_en), Subsystem1/1(sat_en)
  cin/1 -> Mux6/2
  sub_en/1 -> Convert/1
  Subsystem/1(r) -> Concat/2
  Concat/1 -> Mux1/2
  Constant/1 -> Concat/1

== system scalar_processor/Integer Multiply 24-bit ==
  a : Inport
  b : Inport  Port=2
  a_neg : Inport  Port=3
  b_neg : Inport  Port=4
  w32 : Inport  Port=5
  is_signed : Inport  Port=6
  Convert : xbsIndex_r4/Convert  arith_type="Signed  (2's comp)"  n_bits=32  bin_pt=0  quantization=Truncate  overflow=Saturate  en=off  latency=0  dbl_ovrd=off  pipeline=off  block_type=convert
      settings: block_version=12.2
  Convert1 : xbsIndex_r4/Convert  arith_type="Signed  (2's comp)"  n_bits=32  bin_pt=0  quantization=Truncate  overflow=Saturate  en=off  latency=0  dbl_ovrd=off  pipeline=off  block_type=convert
      settings: block_version=12.2
  Mult : xbsIndex_r4/Mult  precision=User Defined  arith_type="Signed  (2's comp)"  n_bits=32  bin_pt=0  quantization=Truncate  overflow=Wrap  en=off  latency=11  dbl_ovrd=off  use_behavioral_HDL=off  opt=Speed  use_embedded=on  optimum_pipeline=on  pipeline=on  use_rpm=on  placement_style=Triangular  block_type=mult
      settings: block_version=12.2
  Mult1 : xbsIndex_r4/Mult  precision=User Defined  arith_type=Unsigned  n_bits=32  bin_pt=0  quantization=Truncate  overflow=Wrap  en=off  latency=11  dbl_ovrd=off  use_behavioral_HDL=off  opt=Speed  use_embedded=on  optimum_pipeline=on  pipeline=on  use_rpm=on  placement_style=Triangular  block_type=mult
      settings: block_version=12.2
  Mux : xbsIndex_r4/Mux  inputs=2  en=off  latency=0  precision=Full  arith_type=Unsigned  n_bits=16  bin_pt=14  quantization=Truncate  overflow=Wrap  dbl_ovrd=off  block_type=mux
      settings: block_version=12.2
  a_signed : Subsystem
  a_unsigned : Subsystem
  b_signed : Subsystem
  b_unsigned : Subsystem
  result : Outport
  wires:
  Convert/1 -> a_signed/3(sgn)
  Convert1/1 -> b_signed/3(sgn)
  a_signed/1(srslt) -> Mult/1
  b_signed/1(srslt) -> Mult/2
  a_unsigned/1(urslt) -> Mult1/1
  b_unsigned/1(urslt) -> Mult1/2
  Mult/1 -> Mux/3
  Mult1/1 -> Mux/2
  Mux/1 -> result/1
  is_signed/1 -> Mux/1
  a/1 -> Convert/1, a_unsigned/3(usgn)
  b/1 -> Convert1/1, b_unsigned/3(usgn)
  a_neg/1 -> a_unsigned/2(neg), a_signed/1(neg)
  b_neg/1 -> b_signed/1(neg), b_unsigned/2(neg)
  w32/1 -> a_signed/2(w32), b_signed/2(w32), a_unsigned/1(w32), b_unsigned/1(w32)

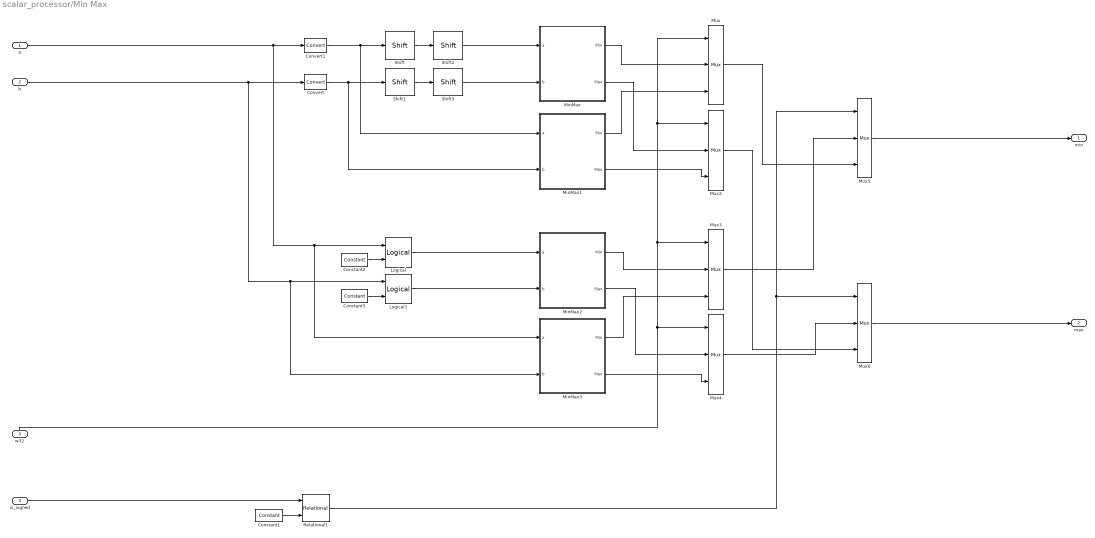
== system scalar_processor/Min Max ==
  a : Inport
  b : Inport  Port=2
  w32 : Inport  Port=3
  is_signed : Inport  Port=4
  Constant1 : xbsIndex_r4/Constant  arith_type=Unsigned  const=1  n_bits=1  bin_pt=0  explicit_period=off  period=1  equ=P=C  opselect=C  inp2=PCIN>>17  opr=+  inp1=P  carry=CIN  dbl_ovrd=off  block_type=constant
      settings: block_version=12.2
  Constant2 : xbsIndex_r4/Constant  arith_type=Unsigned  const=65535  n_bits=32  bin_pt=0  explicit_period=off  period=1  equ=P=C  opselect=C  inp2=PCIN>>17  opr=+  inp1=P  carry=CIN  dbl_ovrd=off  block_type=constant
      settings: block_version=12.2
  Constant3 : xbsIndex_r4/Constant  arith_type=Unsigned  const=65535  n_bits=32  bin_pt=0  explicit_period=off  period=1  equ=P=C  opselect=C  inp2=PCIN>>17  opr=+  inp1=P  carry=CIN  dbl_ovrd=off  block_type=constant
      settings: block_version=12.2
  Convert : xbsIndex_r4/Convert  arith_type="Signed  (2's comp)"  n_bits=31  bin_pt=0  quantization=Truncate  overflow=Saturate  en=off  latency=0  dbl_ovrd=off  pipeline=off  block_type=convert
      settings: block_version=12.2
  Convert1 : xbsIndex_r4/Convert  arith_type="Signed  (2's comp)"  n_bits=32  bin_pt=0  quantization=Truncate  overflow=Saturate  en=off  latency=0  dbl_ovrd=off  pipeline=off  block_type=convert
      settings: block_version=12.2
  Logical : xbsIndex_r4/Logical  logical_function=AND  inputs=2  en=off  latency=0  precision=User Defined  arith_type=Unsigned  n_bits=32  bin_pt=0  align_bp=on  dbl_ovrd=off  block_type=logical
      settings: block_version=12.2
  Logical1 : xbsIndex_r4/Logical  logical_function=AND  inputs=2  en=off  latency=0  precision=User Defined  arith_type=Unsigned  n_bits=32  bin_pt=0  align_bp=on  dbl_ovrd=off  block_type=logical
      settings: block_version=12.2
  MinMax : Subsystem
  MinMax1 : Subsystem
  MinMax2 : Subsystem
  MinMax3 : Subsystem
  Mux{,2..4} (4 alike) : xbsIndex_r4/Mux  inputs=2  en=off  latency=0  precision=Full  arith_type=Unsigned  n_bits=16  bin_pt=14  quantization=Truncate  overflow=Wrap  dbl_ovrd=off  block_type=mux
      settings: block_version=12.2
  Mux5 : xbsIndex_r4/Mux  inputs=2  en=off  latency=0  precision=User Defined  arith_type="Signed  (2's comp)"  n_bits=32  bin_pt=0  quantization=Truncate  overflow=Saturate  dbl_ovrd=off  block_type=mux
      settings: block_version=12.2
  Mux6 : xbsIndex_r4/Mux  inputs=2  en=off  latency=0  precision=User Defined  arith_type=Unsigned  n_bits=32  bin_pt=0  quantization=Truncate  overflow=Saturate  dbl_ovrd=off  block_type=mux
      settings: block_version=12.2
  Relational1 : xbsIndex_r4/Relational  mode=a=b  en=off  latency=0  dbl_ovrd=off  block_type=relational
      settings: block_version=12.2
  Shift : xbsIndex_r4/Shift  shift_dir=Left  shift_bits=16  en=off  latency=0  precision=Full  arith_type="Signed  (2's comp)"  n_bits=31  bin_pt=0  quantization=Truncate  overflow=Saturate  dbl_ovrd=off  block_type=shift
      settings: block_version=12.2
  Shift1 : xbsIndex_r4/Shift  shift_dir=Left  shift_bits=16  en=off  latency=0  precision=Full  arith_type="Signed  (2's comp)"  n_bits=31  bin_pt=0  quantization=Truncate  overflow=Saturate  dbl_ovrd=off  block_type=shift
      settings: block_version=12.2
  Shift2 : xbsIndex_r4/Shift  shift_dir=Right  shift_bits=16  en=off  latency=0  precision=Full  arith_type="Signed  (2's comp)"  n_bits=31  bin_pt=0  quantization=Truncate  overflow=Saturate  dbl_ovrd=off  block_type=shift
      settings: block_version=12.2
  Shift3 : xbsIndex_r4/Shift  shift_dir=Right  shift_bits=16  en=off  latency=0  precision=Full  arith_type="Signed  (2's comp)"  n_bits=31  bin_pt=0  quantization=Truncate  overflow=Saturate  dbl_ovrd=off  block_type=shift
      settings: block_version=12.2
  min : Outport
  max : Outport  Port=2
  wires:
  Constant1/1 -> Relational1/2
  b/1 -> Convert/1, Logical1/1, MinMax3/2(b)
  a/1 -> Convert1/1, Logical/1, MinMax3/1(a)
  Convert1/1 -> Shift/1, MinMax1/1(a)
  Convert/1 -> Shift1/1, MinMax1/2(b)
  Shift1/1 -> Shift3/1
  Shift/1 -> Shift2/1
  Shift2/1 -> MinMax/1(a)
  Shift3/1 -> MinMax/2(b)
  w32/1 -> Mux/1, Mux2/1, Mux3/1, Mux4/1
  MinMax/1(Min) -> Mux/2
  MinMax1/1(Min) -> Mux/3
  MinMax/2(Max) -> Mux2/2
  MinMax1/2(Max) -> Mux2/3
  Constant2/1 -> Logical/2
  Constant3/1 -> Logical1/2
  Logical/1 -> MinMax2/1(a)
  Logical1/1 -> MinMax2/2(b)
  MinMax2/1(Min) -> Mux3/2
  MinMax3/1(Min) -> Mux3/3
  MinMax2/2(Max) -> Mux4/2
  MinMax3/2(Max) -> Mux4/3
  Relational1/1 -> Mux5/1, Mux6/1
  Mux/1 -> Mux5/3
  Mux2/1 -> Mux6/3
  Mux3/1 -> Mux5/2
  Mux4/1 -> Mux6/2
  Mux5/1 -> min/1
  Mux6/1 -> max/1
  is_signed/1 -> Relational1/1

== system scalar_processor/Shift Logical ==
  a : Inport
  b : Inport  Port=2
  w32 : Inport  Port=3
  is_signed : Inport  Port=4
  Slice : xbsIndex_r4/Slice  nbits=5  boolean_output=off  mode=Lower Bit Location + Width  bit1=0  base1=MSB of Input  bit0=0  base0=LSB of Input  dbl_ovrd=off  block_type=slice
  sll : Subsystem
  sll_select : Subsystem
  srl : Subsystem
  srl_select : Subsystem
  shift_left : Outport
  shift_right : Outport  Port=2
  wires:
  Slice/1 -> srl/1(srl_amt), sll/1(sll_amt)
  sll/1(sll_out) -> sll_select/2(sll_in)
  sll_select/1(sll_out) -> shift_left/1
  srl/1(srl_out) -> srl_select/5(srl_in)
  srl_select/1(srl_out) -> shift_right/1
  b/1 -> Slice/1, sll_select/1(b), srl_select/2(b)
  a/1 -> sll/2(a), srl/2(a), srl_select/1(a)
  w32/1 -> sll_select/3(w32), srl/4(w32), srl_select/3(w32)
  is_signed/1 -> srl/3(is_signed), srl_select/4(is_signed)
